simulink model "mayatnik"  (R2015b)
settings: Solver=ode45  StartTime=0.0  StopTime=500  MaxStep=0.01  RelTol=1e-3
undefined symbols (not defined in the file): A1, A2, F1, F2max, g, l, m, Omega, x0
libraries: simulink x3
settings Model: Creator=DNikolaev  LastModifiedBy=DNikolaev

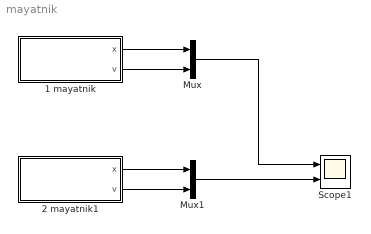
== system mayatnik ==
  1 mayatnik : Subsystem
  2 mayatnik1 : Subsystem
  Mux : Mux  Inputs=2
  Mux1 : Mux  Inputs=2
  Scope1 : Scope  NumInputPorts=2
  wires:
  1 mayatnik/1(x) -> Mux/1
  1 mayatnik/2(v) -> Mux/2
  Mux/1 -> Scope1/1
  2 mayatnik1/1(x) -> Mux1/1
  2 mayatnik1/2(v) -> Mux1/2
  Mux1/1 -> Scope1/2

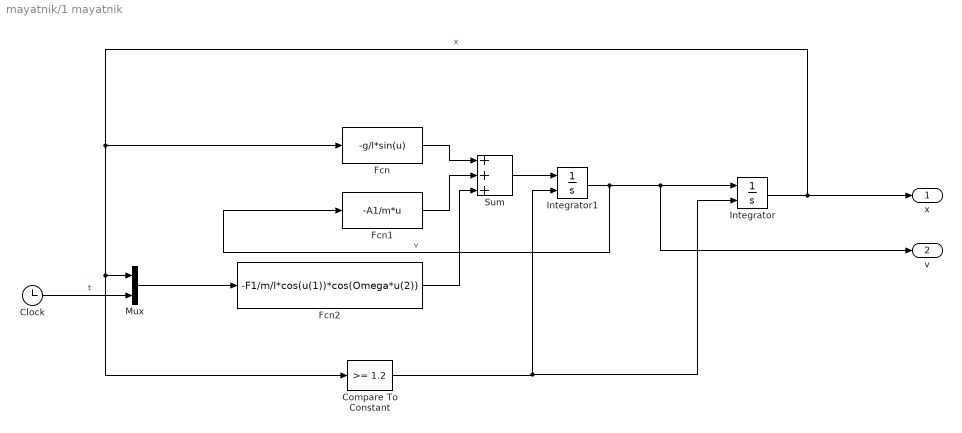
== system mayatnik/1 mayatnik ==
  Clock : Clock
  Compare To Constant : simulink/Logic and Bit Operations/Compare To Constant  relop=>=  const=1.2  OutDataTypeStr=boolean
  Fcn : Fcn  Expr=-g/l*sin(u)
  Fcn1 : Fcn  Expr=-A1/m*u
  Fcn2 : Fcn  Expr=-F1/m/l*cos(u(1))*cos(Omega*u(2))
  Integrator : Integrator  ExternalReset=level  InitialCondition=x0
  Integrator1 : Integrator  ExternalReset=level
  Mux : Mux  Inputs=2
  Sum : Sum  Inputs=+++
  x : Outport
  v : Outport  Port=2
  wires:
  Integrator/1 -> Fcn/1, Compare To Constant/1, Mux/1, x/1  "x"
  Integrator1/1 -> v/1, Integrator/1, Fcn1/1  "v"
  Mux/1 -> Fcn2/1
  Clock/1 -> Mux/2  "t"
  Sum/1 -> Integrator1/1
  Fcn1/1 -> Sum/2
  Fcn/1 -> Sum/1
  Fcn2/1 -> Sum/3
  Compare To Constant/1 -> Integrator/2, Integrator1/2

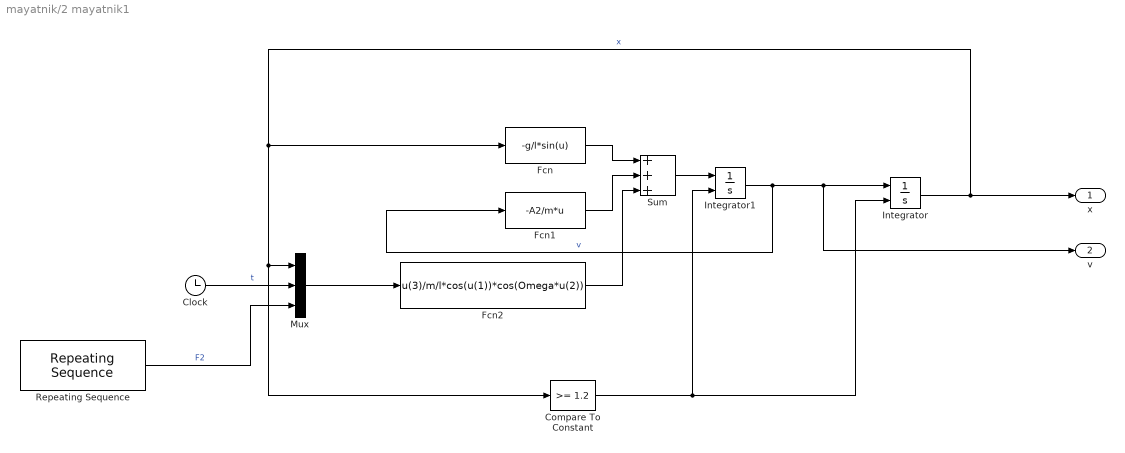
== system mayatnik/2 mayatnik1 ==
  Clock : Clock
  Compare To Constant : simulink/Logic and Bit Operations/Compare To Constant  relop=>=  const=1.2  OutDataTypeStr=boolean
  Fcn : Fcn  Expr=-g/l*sin(u)
  Fcn1 : Fcn  Expr=-A2/m*u
  Fcn2 : Fcn  Expr=u(3)/m/l*cos(u(1))*cos(Omega*u(2))
  Integrator : Integrator  ExternalReset=level  InitialCondition=x0
  Integrator1 : Integrator  ExternalReset=level
  Mux : Mux  Inputs=3
  Repeating Sequence : simulink/Sources/Repeating Sequence  rep_seq_t=[0 10 20]  rep_seq_y=[0 F2max 0]
  Sum : Sum  Inputs=+++
  x : Outport
  v : Outport  Port=2
  wires:
  Fcn2/1 -> Sum/3
  Fcn/1 -> Sum/1
  Fcn1/1 -> Sum/2
  Sum/1 -> Integrator1/1
  Clock/1 -> Mux/2  "t"
  Mux/1 -> Fcn2/1
  Integrator1/1 -> Integrator/1, v/1, Fcn1/1  "v"
  Integrator/1 -> Compare To Constant/1, Mux/1, Fcn/1, x/1  "x"
  Repeating Sequence/1 -> Mux/3  "F2"
  Compare To Constant/1 -> Integrator/2, Integrator1/2
